simulink model "modello"  (R2014a)
settings: Solver=ode45  StartTime=0.0  StopTime=100.0  RelTol=1e-3
values from neighbouring files (symbols this model uses):
  masses = [m1;m2;m3]    [init.m]    (also in parinit.m; trajectory_tvp.m)
  nq = 3    [init.m]    (also in parinit.m)
  q0 = rand(nq,1)    [init.m]    (also in parinit.m = [0,deg2rad(90),1])
  qp0 = zeros(nq,1)    [init.m]    (also in parinit.m = [1;0;0])
settings Model: Creator=danilo  LastModifiedBy=danilo

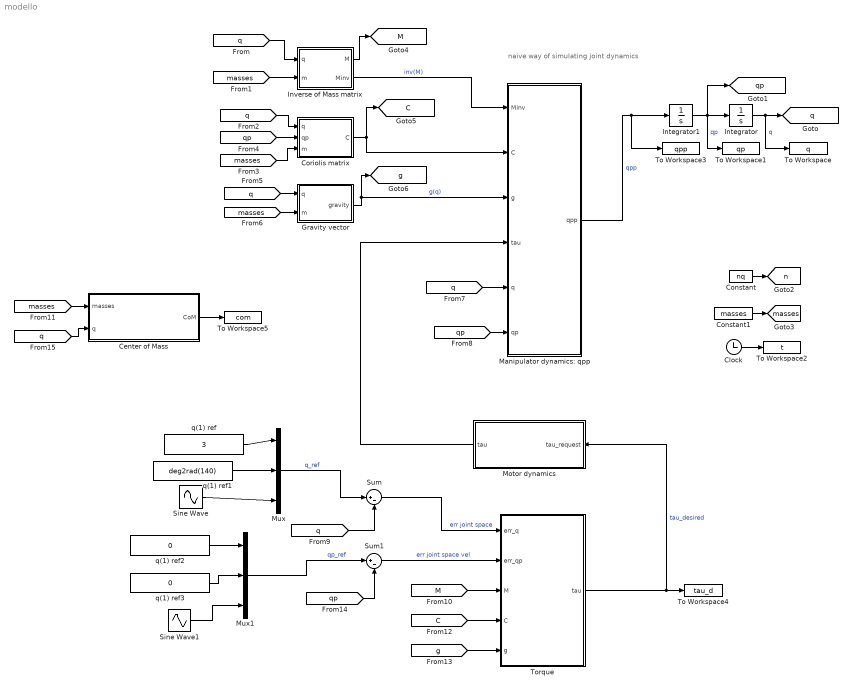
== system modello ==
  note: naive way of simulating joint dynamics
  Center of Mass : MATLAB Function  TreatAsAtomicUnit=on
  Clock : Clock
  Constant : Constant  Value=nq
  Constant1 : Constant  Value=masses
  Coriolis matrix : MATLAB Function  TreatAsAtomicUnit=on
  Gravity vector : MATLAB Function  TreatAsAtomicUnit=on
  Integrator : Integrator  InitialCondition=q0
  Integrator1 : Integrator  InitialCondition=qp0
  Inverse of Mass matrix : MATLAB Function  TreatAsAtomicUnit=on
  Manipulator dynamics: qpp : MATLAB Function  TreatAsAtomicUnit=on
  Motor dynamics : MATLAB Function  TreatAsAtomicUnit=on
  Mux : Mux  Inputs=3
  Mux1 : Mux  Inputs=3
  Sine Wave : Sin  Bias=5  SampleTime=0
  Sine Wave1 : Sin  Bias=1.5  Phase=pi/2  SampleTime=0
  Sum : Sum  Inputs=|+-
  Sum1 : Sum  Inputs=|+-
  To Workspace : ToWorkspace  VariableName=q  SampleTime=-1
  To Workspace1 : ToWorkspace  VariableName=qp  SampleTime=-1
  To Workspace2 : ToWorkspace  VariableName=t  SampleTime=-1
  To Workspace3 : ToWorkspace  VariableName=qpp  SampleTime=-1
  To Workspace4 : ToWorkspace  VariableName=tau_d  SampleTime=-1
  To Workspace5 : ToWorkspace  VariableName=com  SampleTime=-1
  Torque : MATLAB Function  TreatAsAtomicUnit=on
  q(1) ref : Constant  Value=3
  q(1) ref1 : Constant  Value=deg2rad(140)
  q(1) ref2 : Constant  Value=0
  q(1) ref3 : Constant  Value=0
  tag scope: C=global, M=global, g=global, masses=global, n=global, q=global, qp=global
  wires:
  Integrator1/1 -> To Workspace1/1, [qp], Integrator/1  "qp"
  Integrator/1 -> To Workspace/1, [q]  "q"
  [q] -> Inverse of Mass matrix/1(q)
  Inverse of Mass matrix/2(Minv) -> Manipulator dynamics: qpp/1(Minv)  "inv(M)"
  Manipulator dynamics: qpp/1(qpp) -> To Workspace3/1, Integrator1/1  "qpp"
  Gravity vector/1(gravity) -> [g], Manipulator dynamics: qpp/3(g)  "g(q)"
  Coriolis matrix/1(C) -> [C], Manipulator dynamics: qpp/2(C)
  Constant/1 -> [n]
  [qp] -> Coriolis matrix/2(qp)
  [q] -> Coriolis matrix/1(q)
  [q] -> Gravity vector/1(q)
  [masses] -> Gravity vector/2(m)
  Torque/1(tau) -> Motor dynamics/1(tau_request), To Workspace4/1  "tau_desired"
  [q] -> Manipulator dynamics: qpp/5(q)
  [qp] -> Manipulator dynamics: qpp/6(qp)
  Constant1/1 -> [masses]
  [masses] -> Inverse of Mass matrix/2(m)
  [masses] -> Coriolis matrix/3(m)
  Clock/1 -> To Workspace2/1
  Mux/1 -> Sum/1  "q_ref"
  [q] -> Sum/2
  Sum/1 -> Torque/1(err_q)  "err joint space"
  Inverse of Mass matrix/1(M) -> [M]
  [M] -> Torque/3(M)
  [C] -> Torque/4(C)
  [g] -> Torque/5(g)
  Mux1/1 -> Sum1/1  "qp_ref"
  [qp] -> Sum1/2
  Sum1/1 -> Torque/2(err_qp)  "err joint space vel"
  Motor dynamics/1(tau) -> Manipulator dynamics: qpp/4(tau)
  q(1) ref/1 -> Mux/1
  Sine Wave/1 -> Mux/3
  q(1) ref1/1 -> Mux/2
  q(1) ref2/1 -> Mux1/1
  Sine Wave1/1 -> Mux1/3
  q(1) ref3/1 -> Mux1/2
  [masses] -> Center of Mass/1(masses)
  [q] -> Center of Mass/2(q)
  Center of Mass/1(CoM) -> To Workspace5/1

== matlab function modello/Coriolis matrix ==
  data: q input; qp input; C output; m input
function C = fcn(q,qp,m)
%#codegen

% C = [0,(-1).*m(3).*(cos(q(2)).*q(3).*qp(2)+sin(q(2)).* ...
%   qp(3)),(-1).*m(3).*sin(q(2)).*qp(2); ...
%   0,m(3).*q(3).*qp(3),m(3).*q(3).*qp(2); ...
%   0,(-1).*m(3).*q(3).*qp(2),0];
%% calcolata a mano da lagrangiana
C = [-2.*m(3).*sin(q(2)).*qp(3).*qp(2)-m(3).*q(3).*cos(q(2)).*qp(2)^2;
    2.*m(3).*q(3).*qp(3).*qp(2)-m(3).*sin(q(2)).*qp(1).*qp(3)-m(3).*q(3).*cos(q(2)).*qp(1).*qp(2);
    -m(3).*sin(q(2)).*qp(1).*qp(2)];

== matlab function modello/Inverse of Mass matrix ==
  data: M output; q input; Minv output; m input
function [M,Minv] = fcn(q,m)
%#codegen

% M inversa
Minv = [m(1).^(-1),m(1).^(-1).*q(3).^(-1).*sin(q(2)),(-1).*m(1).^(-1).*cos( ...
  q(2));m(1).^(-1).*q(3).^(-1).*sin(q(2)),m(1).^(-1).*m(3).^(-1).*(m(1)+ ...
  m(3)+(-1).*m(3).*cos(q(2)).^2).*q(3).^(-2),(-1).*m(1).^(-1).*cos(q(2) ...
  ).*q(3).^(-1).*sin(q(2));(-1).*m(1).^(-1).*cos(q(2)),(-1).*m(1).^( ...
  -1).*cos(q(2)).*q(3).^(-1).*sin(q(2)),m(1).^(-1).*m(3).^(-1).*(m(1)+ ...
  m(3)+(-1).*m(3).*sin(q(2)).^2)];

% M non invertita
M = [m(1)+m(3),(-1).*m(3).*q(3).*sin(q(2)),m(3).*cos(q(2));(-1).*m(3).*q(3) ...
   .*sin(q(2)),m(3).*q(3).^2,0;m(3).*cos(q(2)),0,m(3)];

== matlab function modello/Gravity vector ==
  data: q input; gravity output; m input
function gravity = fcn(q,m)
%#codegen
g = 9.81;
% gravity = [0,0,0];
%% calcolato a mano da lagrangiana
gravity = [0;-m(3).*g.*q(3).*cos(q(2));
    m(3).*g.*sin(q(2))];

== matlab function modello/Torque ==
  data: err_q input; err_qp input; tau output; M input; C input; g input
function tau = fcn(err_q,err_qp,M,C,g)
%#codegen

tau = zeros(3,1);
tau(1) = 10;
tau(3) = 10;

qref = [1;0;2];
compensate = g+C;
u = eye(3)*err_q + eye(3)*err_qp;
KP_cart = eye(2);
KP_pend = 1;
KP = blkdiag(KP_cart,KP_pend);
KD_cart = eye(2);
KD_pend = 1;
KD = blkdiag(KD_cart,KD_pend);
u = KP*err_q + KD*err_qp;
control = M*(u);
tau = compensate + control;
% tau(2)=0;

== matlab function modello/Manipulator dynamics: qpp ==
  data: Minv input; C input; g input; tau input; q input; qp input; qpp output
function qpp = fcn(Minv,C,g, tau,q,qp)
%#codegen
g = g(:); % column
% qpp = -Minv*(C*qp+g-tau);
%% da lagrangiana
qpp = -Minv*(C+g-tau);

== matlab function modello/Motor dynamics ==
  data: tau_request input; tau output
function tau = fcn(tau_request)
%#codegen

% here we could insert the walkman
% actuator dynamics
tau = tau_request;

== matlab function modello/Center of Mass ==
  data: masses input; CoM output; q input
function CoM = fcn(masses,q)
%#codegen
% q = [cart position, pendulum angle, pendulum length];
px = q(1) + q(3).*cos(q(2));
positions = [q(1), q(2), px];
CoM = dot(masses,positions)/sum(masses);
